simulink model "finalproject2"  (R2017a)
settings: Solver=VariableStepAuto  StartTime=0.0  StopTime=10.0  RelTol=1e-3
settings Model: Creator=xiaodong  LastModifiedBy=xiaodong

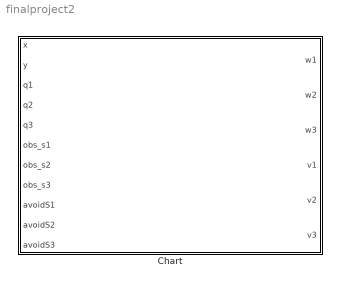
== system finalproject2 ==
  Chart : Stateflow chart  TreatAsAtomicUnit=on

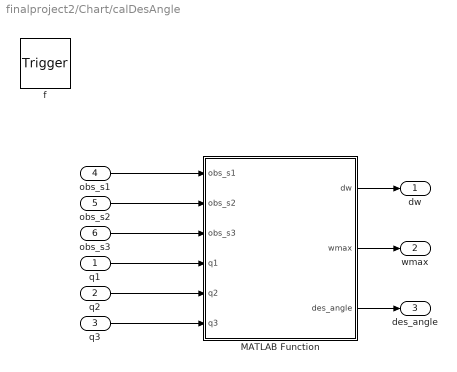
== system finalproject2/Chart/calDesAngle ==
  q1 : Inport  OutDataTypeStr=double  PortDimensions=1
  q2 : Inport  Port=2  OutDataTypeStr=double  PortDimensions=1
  q3 : Inport  Port=3  OutDataTypeStr=double  PortDimensions=1
  obs_s1 : Inport  Port=4  OutDataTypeStr=double  PortDimensions=1
  obs_s2 : Inport  Port=5  OutDataTypeStr=double  PortDimensions=1
  obs_s3 : Inport  Port=6  OutDataTypeStr=double  PortDimensions=1
  f : TriggerPort  TriggerType=function-call  VariantControl=Variant
      settings: CopyFcn=Stateflow.SLINSF.SimulinkMan.removeBlockPreDeleteFcn  PreDeleteFcn=Stateflow.SLINSF.SimulinkMan.unsafePredeleteFcn
  MATLAB Function : MATLAB Function  TreatAsAtomicUnit=on
  dw : Outport
  wmax : Outport  Port=2
  des_angle : Outport  Port=3
  wires:
  obs_s1/1 -> MATLAB Function/1(obs_s1)
  obs_s2/1 -> MATLAB Function/2(obs_s2)
  obs_s3/1 -> MATLAB Function/3(obs_s3)
  MATLAB Function/3(des_angle) -> des_angle/1
  MATLAB Function/1(dw) -> dw/1
  MATLAB Function/2(wmax) -> wmax/1
  q1/1 -> MATLAB Function/4(q1)
  q2/1 -> MATLAB Function/5(q2)
  q3/1 -> MATLAB Function/6(q3)

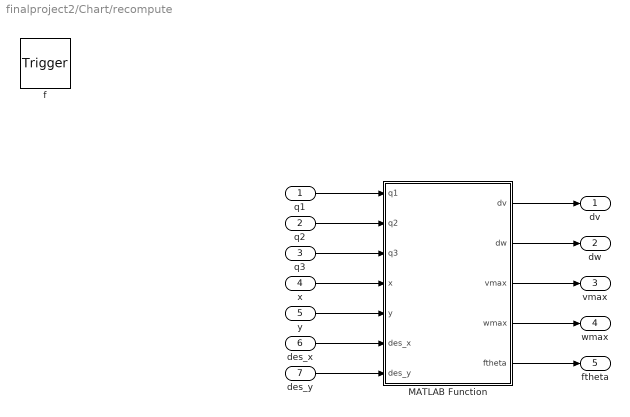
== system finalproject2/Chart/recompute ==
  q1 : Inport  OutDataTypeStr=double  PortDimensions=1
  q2 : Inport  Port=2  OutDataTypeStr=double  PortDimensions=1
  q3 : Inport  Port=3  OutDataTypeStr=double  PortDimensions=1
  x : Inport  Port=4  OutDataTypeStr=double  PortDimensions=1
  y : Inport  Port=5  OutDataTypeStr=double  PortDimensions=1
  des_x : Inport  Port=6  OutDataTypeStr=double  PortDimensions=1
  des_y : Inport  Port=7  OutDataTypeStr=double  PortDimensions=1
  f : TriggerPort  TriggerType=function-call  VariantControl=Variant
      settings: CopyFcn=Stateflow.SLINSF.SimulinkMan.removeBlockPreDeleteFcn  PreDeleteFcn=Stateflow.SLINSF.SimulinkMan.unsafePredeleteFcn
  MATLAB Function : MATLAB Function  TreatAsAtomicUnit=on
  dv : Outport
  dw : Outport  Port=2
  vmax : Outport  Port=3
  wmax : Outport  Port=4
  ftheta : Outport  Port=5
  wires:
  MATLAB Function/1(dv) -> dv/1
  MATLAB Function/2(dw) -> dw/1
  MATLAB Function/3(vmax) -> vmax/1
  MATLAB Function/4(wmax) -> wmax/1
  y/1 -> MATLAB Function/5(y)
  q1/1 -> MATLAB Function/1(q1)
  x/1 -> MATLAB Function/4(x)
  des_x/1 -> MATLAB Function/6(des_x)
  q2/1 -> MATLAB Function/2(q2)
  q3/1 -> MATLAB Function/3(q3)
  des_y/1 -> MATLAB Function/7(des_y)
  MATLAB Function/5(ftheta) -> ftheta/1

== matlab function finalproject2/Chart/calDesAngle/MATLAB Function ==
  data: dw output; wmax output; obs_s1 input; obs_s2 input; obs_s3 input; des_angle output; q1 input; q2 input; q3 input
function [dw, wmax, des_angle] = calDesAngle(obs_s1, obs_s2, obs_s3, q1, q2, q3)
 
    obs_angle1 = obs_s1(1);
    obs_dist1 = obs_s1(2);
    
    obs_angle2 = obs_s2(1);
    obs_dist2 = obs_s2(2);
    if( obs_dist1 <= obs_dist2 )
        main_angle = obs_angle1; 
    else
        main_angle = obs_angle2;
    end
    
    if(abs(main_angle) < 1.0)
        if(main_angle > 0)
            des_angle = main_angle - M_PI /1.8;
        else
            des_angle = pi /1.8 - main_angle;
        end

    elseif(fabs(main_angle) > 1.0 )
        des_angle = 0;
    end
    
    curent_orientation1 = 2 * atan2(q1(1), q1(2));
    curent_orientation2 = 2 * atan2(q2(1), q2(2));
    curent_orientation3 = 2 * atan2(q3(1), q3(2));
    
    relative1 = des_theta - curent_orientation1;
    relative2 = des_theta - curent_orientation2;
    relative3 = des_theta - curent_orientation3;
    
    delta_t = 50;
    wmax1 = 2 * relative1 / delta_t;
    dw1 = 2 * wmax1 / delta_t;
    
    wmax2 = 2 * relative2 / delta_t;
    dw2 = 2 * wmax2 / delta_t;
    
    wmax3 = 2 * relative3 / delta_t;
    dw3 = 2 * wmax3 / delta_t;
    
    dw = [dw1; dw2; dw3];
    wmax = [wmax1; wmax2; wmax3];
end

== matlab function finalproject2/Chart/recompute/MATLAB Function ==
  data: q1 input; q2 input; q3 input; x input; y input; des_x input; des_y input; dv output; dw output; vmax output; wmax output; ftheta output
function [dv, dw,vmax, wmax, ftheta] = recompute(q1, q2, q3, x, y, des_x, des_y)
    cur_x1 = x(1);  cur_x2 = x(2); cur_x3 = x(3);
    cur_y1 = y(1);  cur_y2 = y(2); cur_y3 = y(3);
    
    des_x1 = des_x(1);  des_x2 = des_x(2); des_x3 = des_x(3);
    des_y1 = des_y(1);  des_y2 = des_y(2); des_y3 = des_y(3);
    
    [twist_1, ftheta1] = pointTopoint(q1, cur_x1, cur_y1, des_x1, des_y1);
    [twist_2, ftheta2] = pointTopoint(q2, cur_x2, cur_y2, des_x2, des_y2);
    [twist_3, ftheta3] = pointTopoint(q3, cur_x3, cur_y3, des_x3, des_y3);
    ftheta = [ftheta1; ftheta2; ftheta3];
    
    v1_max = twist_1(0);
    v2_max = twist_2(0);
    v3_max = twist_3(0);
    vmax = [v1_max; v2_max; v3_max];
    
    w1_max = twist_1(1);
    w2_max = twist_2(1);
    w3_max = twist_3(1);
    wmax = [w1_max; w2_max; w3_max];
    
    delta_speed1 = 2 * v1_max / delta_t; 
    delta_speed2 = 2 * v2_max / delta_t;
    delta_speed3 = 2 * v3_max / delta_t;

    delta_w1 = 2 * w1_max / delta_t; //spped steps
    delta_w2 = 2 * w2_max / delta_t;
    delta_w3 = 2 * w3_max / delta_t;
    
    dv = [delta_speed1; delta_speed2; delta_speed3];
    dw = [delta_w1; delta_w2; delta_w3]; 
end

function [twist_max, ftheta]= pointTopoint(q, cur_x, cur_y, des_x, des_y)
    twist_max = [];
    delta_x = des_x - cur_x;
    delta_y = des_y - cur_y;
    des_theta = atan2(delta_y, delta_x);
    ftheta = des_theta;
    travel_dist = delta_x / cos(des_theta);
    
    qz = q(1); qw = q(2);
    curent_orientation = 2 * atan2(qz, qw);
    
    relative_theta = des_theta - curent_orientation;
    w_max = 2 * relative_theta / delta_t;
    vx_max = 2 * travel_dist / delta_t;
    twist_max(0) = vx_max;
    twist_max(1) = w_max;
end

== stateflow chart finalproject2/Chart ==
  settings: updateMethod=CONTINUOUS
  state [dv, dw,vmax, wmax, ftheta] = recompute(q1, q2, q3, x, y, des_x, des_y) [function]
  state [dw,wmax,des_angle] = calDesAngle(q1,q2,q3,obs_s1,obs_s2,obs_s3) [function]
  state reschedule
    state reorient
      during:
      w1_dot = dw(1); w2_dot = dw(2); w3_dot = dw(3);
      theta1_dot = w1; theta2_dot = w2;  theta3_dot = w3;
    state recompute
      entry:
      [dv, dw,vmax, wmax, ftheta] =...
      recompute(q1, q2, q3, x, y, des_x, des_y);
    reorient -> reorient [order 2] : [abs(theta1 - ftheta(1))<=thresht&&flag1 == 0]{dw(1) = 0; w1 = 0; flag1 = 1;}
    reorient -> reorient [order 1] : [abs(theta2 - ftheta(2))<=thresht&&flag2 == 0]{dw(2) = 0; w2 = 0; flag2 = 1;}
    reorient -> reorient [order 3] : [abs(theta3 - ftheta(3))<=thresht && flag3 == 0]{dw(3) = 0; w3 = 0;flag3 =1;}
    (default) -> recompute
    recompute -> reorient : {flag1 = 0; flag2 = 0; flag3 = 0;...
        | v1 = 0; v2 = 0; v3 = 0;}
    reorient -> reorient [order 4] : [abs(w1-wmax(1))<=threshw]{dw(1) = -dw(1);}
    reorient -> reorient [order 6] : [abs(w2-wmax(2))<=threshw]{dw(2) = -dw(2);}
    reorient -> reorient [order 5] : [abs(w3-wmax(3))<=threshw]{dw(3) = -dw(3);}
  state goToPosition
    during:
    v1_dot = dv(1);  v2_dot = dv(2);  v3_dot = dv(3);
    deltax1_dot = v1;  deltax2_dot = v2; deltax3_dot = v3;
  state end
    entry:
    dv(1) = 0; dv(2) = 0; dv(3) = 0;
    dw(1) =0; dw(2) = 0; dw(3) = 0;
    w1 = 0; w2 = 0; w3 = 0;
    v1 = 0; v2 = 0; v3 = 0;
  state AvoidController
    state Des_Angle
      state Calculate_Des_Angle
        entry:
        [dv, dw,vmax, wmax, ftheta] =...
        calDesAngle(q1, q2, q3, obs_s1, obs_s2, obs_s3);
      state Turn_Angle
        during:
        w1_dot = dw(1); w2_dot = dw(2); w3_dot = dw(3);
        theta1_dot = w1; theta2_dot = w2;  theta3_dot = w3;
      (default) -> Calculate_Des_Angle
      Calculate_Des_Angle -> Turn_Angle : {flag1 = 0; flag2 = 0; flag3 = 0;}
      Turn_Angle -> Turn_Angle [order 2] : [abs(theta1 - ftheta(1))<=thresht&&flag1 == 0]{dw(1) = 0; w1 = 0; flag1 = 1;}
      Turn_Angle -> Turn_Angle [order 1] : [abs(theta2 - ftheta(2))<=thresht&&flag2 == 0]{dw(2) = 0; w2 = 0; flag2 = 1;}
      Turn_Angle -> Turn_Angle [order 3] : [abs(theta3 - ftheta(3))<=thresht && flag3 == 0]{dw(3) = 0; w3 = 0;flag3 =1;}
      Turn_Angle -> Turn_Angle [order 4] : [abs(w1-wmax(1))<=threshw]{dw(1) = -dw(1);}
      Turn_Angle -> Turn_Angle [order 6] : [abs(w2-wmax(2))<=threshw]{dw(2) = -dw(2);}
      Turn_Angle -> Turn_Angle [order 5] : [abs(w3-wmax(3))<=threshw]{dw(3) = -dw(3);}
    state Go_Avoiding
      entry:
      dv(1) = 0; dv(2) = 0; dv(3) = 0;
      dw(1) =0; dw(2) = 0; dw(3) = 0;
      w1 = 0; w2 = 0; w3 = 0;
      v1 = 0.2; v2 = 0.2; v3 = 0.2;
      during:
      deltax1_dot = v1; deltax2_dot = v2; deltax3_dot = v3;
    (default) -> Des_Angle : {dv(1) = 0; dv(2) = 0; dv(3) = 0;
        | dw(1) =0; dw(2) = 0; dw(3) = 0;
        | w1 = 0; w2 = 0; w3 = 0;
        | v1 = 0; v2 = 0; v3 = 0;}
    Go_Avoiding -> Des_Angle : [avoidS1 || avoidS2 || avoidS3]{v1 = 0; v2 = 0; v3 = 0;}
    Des_Angle -> Go_Avoiding : [flag1 == 1&&flag2 ==1 && flag3 ==1]
  state Extra_Go
    entry:
    count = 0;
    during:
    deltax1_dot = v1; deltax2_dot = v2;
    deltax3_dot = v3;
    count = count+1;
  (default) -> reschedule
  goToPosition -> goToPosition [order 5] : [abs(x(2)+deltax2 - des_x(2))<=threshd && flag5 == 0]{dv(2) = 0; v2 = 0; flag5 = 1; deltax2 = 0;}
  goToPosition -> goToPosition [order 6] : [abs(x(3)+deltax3 - des_x(3))<=threshd && flag6 ==0]{dv(3) = 0; v3 = 0; flag6 = 1; deltax3 = 0;}
  goToPosition -> goToPosition [order 4] : [abs(x(1)+deltax1 - des_x(1))<=threshd && flag4 == 0]{dv(1) = 0; v1 = 0; flag4 = 1; deltax1 = 0;}
  goToPosition -> end [order 7] : [flag4 == 1&&flag5 ==1 && flag6 ==1]
  reschedule -> goToPosition : [flag1 == 1&&flag2 ==1 && flag3 ==1]{...
      | flag4 = 0; flag5 = 0; flag6 = 0;}
  goToPosition -> AvoidController [order 8] : [avoidS1 || avoidS2 || avoidS3]
  goToPosition -> goToPosition [order 1] : [abs(v1-vmax(1))<=threshv]{dv(1) = -dv(1);}
  goToPosition -> goToPosition [order 2] : [abs(v2-vmax(2))<=threshv]{dv(2) = -dv(2);}
  goToPosition -> goToPosition [order 3] : [abs(v3-vmax(3))<=threshv]{dv(3) = -dv(3);}
  Extra_Go -> reschedule : [count >=1000]
  AvoidController -> Extra_Go : [~avoidS1 && ~avoidS2 && ~avoidS3]
  data: q1 function_input double size=1; q2 function_input double size=1; q3 function_input double size=1; x function_input double size=1; y function_input double size=1; des_x function_input double size=1; des_y function_input double size=1; dv function_output; dw function_output; vmax function_output; wmax function_output; ftheta function_output; q1 function_input double size=1; q2 function_input double size=1; q3 function_input double size=1; dw function_output; wmax function_output; obs_s1 function_input double size=1; obs_s2 function_input double size=1; obs_s3 function_input double size=1; des_angle function_output; dv local size=3 =[0;0;0]; dw local size=3 =[0;0;0]; vmax local =0; wmax local =0; ftheta local size=3 =[0;0;0]; x input; y input; q1 input; q2 input; q3 input; des_x constant double =50; des_y constant double =50; w1 output; w2 output; w3 output; theta1 local =0; theta2 local =0; theta3 local =0; thresht constant double =0.005; flag1 local =0; flag2 local =0; flag3 local =0; v1 output; v2 output; v3 output; threshw constant double =0.005; deltax1 local; deltax2 local; deltax3 local; threshv constant double =0.005; threshd constant double =0.005; flag4 local =0; flag5 local =0; flag6 local =0; obs_s1 input size=2; obs_s2 input size=2; obs_s3 input size=2; avoidS1 input; avoidS2 input; avoidS3 input; count local
  data w1 settings: updateMethod=SF_CONTINUOUS_TIME_DATA
  data w2 settings: updateMethod=SF_CONTINUOUS_TIME_DATA
  data w3 settings: updateMethod=SF_CONTINUOUS_TIME_DATA
  data theta1 settings: updateMethod=SF_CONTINUOUS_TIME_DATA
  data theta2 settings: updateMethod=SF_CONTINUOUS_TIME_DATA
  data theta3 settings: updateMethod=SF_CONTINUOUS_TIME_DATA
  data v1 settings: updateMethod=SF_CONTINUOUS_TIME_DATA
  data v2 settings: updateMethod=SF_CONTINUOUS_TIME_DATA
  data v3 settings: updateMethod=SF_CONTINUOUS_TIME_DATA
  data deltax1 settings: updateMethod=SF_CONTINUOUS_TIME_DATA
  data deltax2 settings: updateMethod=SF_CONTINUOUS_TIME_DATA
  data deltax3 settings: updateMethod=SF_CONTINUOUS_TIME_DATA
